simulink model "MeUn_VD"  (R2016b)
settings: configuration reference "CodeGenConfigSet" (kept outside this file)
values from neighbouring files (symbols this model uses):
  MeUn_bCrntClsdCtl_C = Calibration.Parameter    [init_MeUn_VD.m]
  MeUn_bFiterAct_C = Calibration.Parameter    [init_MeUn_VD.m]
  MeUn_bFuelTFit_C = Calibration.Parameter    [init_MeUn_VD.m]
  MeUn_CrntCtlIKi_C = Calibration.Parameter    [init_MeUn_VD.m]
  MeUn_CrntCtlIKiNeg_C = Calibration.Parameter    [init_MeUn_VD.m]
  MeUn_CrntCtlIKiPos_C = Calibration.Parameter    [init_MeUn_VD.m]
  MeUn_CrntCtlIWinNeg_C = Calibration.Parameter    [init_MeUn_VD.m]
  MeUn_CrntCtlIWinPos_C = Calibration.Parameter    [init_MeUn_VD.m]
  MeUn_facCrntCtlInit_CUR = Calibration.Parameter    [init_MeUn_VD.m]
  MeUn_facCrntCtlInit_CURX = Calibration.Parameter    [init_MeUn_VD.m]
  MeUn_facCrntCtlMax_C = Calibration.Parameter    [init_MeUn_VD.m]
  MeUn_facCrntCtlMin_C = Calibration.Parameter    [init_MeUn_VD.m]
  MeUn_facCrntOpenCtl_CUR = Calibration.Parameter    [init_MeUn_VD.m]
  MeUn_facCrntOpenCtl_CURX = Calibration.Parameter    [init_MeUn_VD.m]
  MeUn_facFlt1PT1_C = Calibration.Parameter    [init_MeUn_VD.m]
  MeUn_facFlt2PT1_C = Calibration.Parameter    [init_MeUn_VD.m]
  MeUn_iCnvFlowRate_CUR = Calibration.Parameter    [init_MeUn_VD.m]
  MeUn_iCnvFlowRate_CURX = Calibration.Parameter    [init_MeUn_VD.m]
  MeUn_iLin_CUR = Calibration.Parameter    [init_MeUn_VD.m]
  MeUn_iLin_CURX = Calibration.Parameter    [init_MeUn_VD.m]
  MeUn_iSetMin_C = Calibration.Parameter    [init_MeUn_VD.m]
  MeUn_stActrCtl_C = Calibration.Parameter    [init_MeUn_VD.m]
  MeUn_swtFrzICtl_C = Calibration.Parameter    [init_MeUn_VD.m]
  MeUn_swtVolt_C = Calibration.Parameter    [init_MeUn_VD.m]
  MeUn_tDefltTemp_C = Calibration.Parameter    [init_MeUn_VD.m]
  MeUn_tiCrntCtlInit_C = Calibration.Parameter    [init_MeUn_VD.m]
  MeUn_tiSRCMaxDefDeb_C = Calibration.Parameter    [init_MeUn_VD.m]
  MeUn_tiSRCMaxOKDeb_C = Calibration.Parameter    [init_MeUn_VD.m]
  MeUn_tiSRCMinDefDeb_C = Calibration.Parameter    [init_MeUn_VD.m]
  MeUn_tiSRCMinOKDeb_C = Calibration.Parameter    [init_MeUn_VD.m]
  MeUn_tTempInitThrsd_C = Calibration.Parameter    [init_MeUn_VD.m]
  MeUn_uSRCMax_C = Calibration.Parameter    [init_MeUn_VD.m]
  MeUn_uSRCMin_C = Calibration.Parameter    [init_MeUn_VD.m]
  MeUn_VoltLin_CUR = Calibration.Parameter    [init_MeUn_VD.m]
  MeUn_VoltLin_CURX = Calibration.Parameter    [init_MeUn_VD.m]
  SigTst_iMeUnCurrent_C = Calibration.Parameter    [init_MeUn_VD.m]
  SigTst_swtMeUnCurrent_C = Calibration.Parameter    [init_MeUn_VD.m]
undefined symbols (not defined in the file or in its folder): MeUn_VD_DT
libraries: CXLib x11, simulink x1
settings Model: Creator=Wollf  LastModifiedBy=liutao
settings ConfigSetRef: SourceLocation=Base Workspace

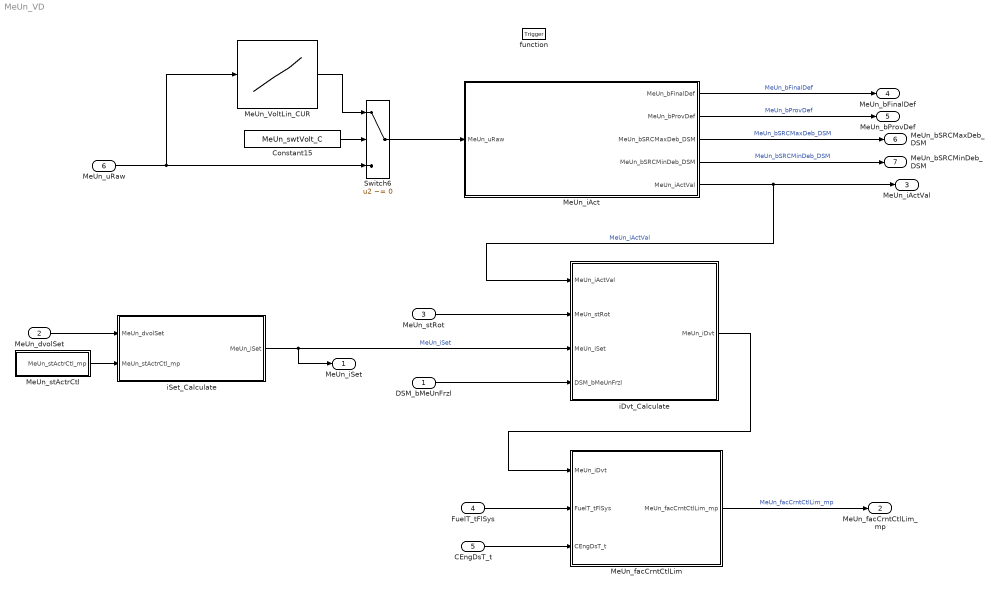
== system MeUn_VD ==
  DSM_bMeUnFrzl : Inport  Description=state of FId_MeUnFrzl  OutMin=0  OutMax=1  OutDataTypeStr=boolean
  MeUn_dvolSet : Inport  Tag=mm^3/s  Description=Setpoint value (volume flow) of rail pressure governing  Port=2  OutMin=-327670  OutMax=327670  OutDataTypeStr=FuelVol_mm3_s
  MeUn_stRot : Inport  Description=State of anchor rotation function of metering unit  Port=3  OutMin=0  OutMax=1  OutDataTypeStr=boolean
  FuelT_tFlSys : Inport  Tag=deg  Description=Fuel system temperature  Port=4  OutMin=-50  OutMax=200  OutDataTypeStr=Temp_deg
  CEngDsT_t : Inport  Tag=deg  Description=engine coolant temperature after filter  Port=5  OutMin=-200  OutMax=200  OutDataTypeStr=Temp_deg
  MeUn_uRaw : Inport  Tag=mv  Description=Raw value of meun  Port=6  OutMin=0  OutMax=5000  OutDataTypeStr=Ad_mv
  function : TriggerPort  TriggerType=function-call  VariantControl=Variant
  Constant15 : Constant  Value=MeUn_swtVolt_C
  MeUn_VoltLin_CUR : Lookup_n-D  NumberOfTableDimensions=1  BreakpointsForDimension1=MeUn_VoltLin_CURX  IndexSearchMethod=Linear search  BeginIndexSearchUsingPreviousIndexResult=on  UseOneInputPortForAllInputData=on  Table=MeUn_VoltLin_CUR  ExtrapMethod=Clip  UseLastTableValue=on  InternalRulePriority=Speed  OutDataTypeStr=Inherit: Inherit via back propagation  SaturateOnIntegerOverflow=on
  MeUn_facCrntCtlLim : Subsystem
  MeUn_iAct : Subsystem
  MeUn_stActrCtl : Subsystem
  Switch6 : Switch  Criteria=u2 ~= 0  InputSameDT=on
  iDvt_Calculate : Subsystem
  iSet_Calculate : Subsystem
  MeUn_iSet : Outport  Tag=mA  Description=Setpoint current for the metering unit  OutMin=-12000  OutMax=12000  OutDataTypeStr=Current_mA
  MeUn_facCrntCtlLim_mp : Outport  Description=Metering unit current control, I component  Port=2  OutMin=0  OutMax=15  OutDataTypeStr=Pid_Kp_Kd
  MeUn_iActVal : Outport  Tag=mA  Description=Current actual value of the analog intput  Port=3  OutMin=-12000  OutMax=12000  OutDataTypeStr=Current_mA
  MeUn_bFinalDef : Outport  Description=the final fault flag  Port=4  OutMin=0  OutMax=1  OutDataTypeStr=boolean
  MeUn_bProvDef : Outport  Description=the fault flag for the moment  Port=5  OutMin=0  OutMax=1  OutDataTypeStr=boolean
  MeUn_bSRCMaxDeb_DSM : Outport  Description=SRC High for metering unit voltage  Port=6  OutMin=0  OutMax=1  OutDataTypeStr=boolean
  MeUn_bSRCMinDeb_DSM : Outport  Description=SRC Low for metering unit voltage  Port=7  OutMin=0  OutMax=1  OutDataTypeStr=boolean
  wires:
  MeUn_stRot/1 -> iDvt_Calculate/2(MeUn_stRot)
  iDvt_Calculate/1(MeUn_iDvt) -> MeUn_facCrntCtlLim/1(MeUn_iDvt)
  MeUn_facCrntCtlLim/1(MeUn_facCrntCtlLim_mp) -> MeUn_facCrntCtlLim_mp/1  "MeUn_facCrntCtlLim_mp"
  DSM_bMeUnFrzl/1 -> iDvt_Calculate/4(DSM_bMeUnFrzl)
  FuelT_tFlSys/1 -> MeUn_facCrntCtlLim/2(FuelT_tFlSys)
  CEngDsT_t/1 -> MeUn_facCrntCtlLim/3(CEngDsT_t)
  Switch6/1 -> MeUn_iAct/1(MeUn_uRaw)
  MeUn_iAct/5(MeUn_iActVal) -> iDvt_Calculate/1(MeUn_iActVal), MeUn_iActVal/1  "MeUn_iActVal"
  MeUn_iAct/1(MeUn_bFinalDef) -> MeUn_bFinalDef/1  "MeUn_bFinalDef"
  MeUn_iAct/2(MeUn_bProvDef) -> MeUn_bProvDef/1  "MeUn_bProvDef"
  MeUn_iAct/3(MeUn_bSRCMaxDeb_DSM) -> MeUn_bSRCMaxDeb_DSM/1  "MeUn_bSRCMaxDeb_DSM"
  MeUn_iAct/4(MeUn_bSRCMinDeb_DSM) -> MeUn_bSRCMinDeb_DSM/1  "MeUn_bSRCMinDeb_DSM"
  iSet_Calculate/1(MeUn_iSet) -> iDvt_Calculate/3(MeUn_iSet), MeUn_iSet/1  "MeUn_iSet"
  MeUn_dvolSet/1 -> iSet_Calculate/1(MeUn_dvolSet)
  MeUn_stActrCtl/1(MeUn_stActrCtl_mp) -> iSet_Calculate/2(MeUn_stActrCtl_mp)
  Constant15/1 -> Switch6/2
  MeUn_uRaw/1 -> MeUn_VoltLin_CUR/1, Switch6/3
  MeUn_VoltLin_CUR/1 -> Switch6/1

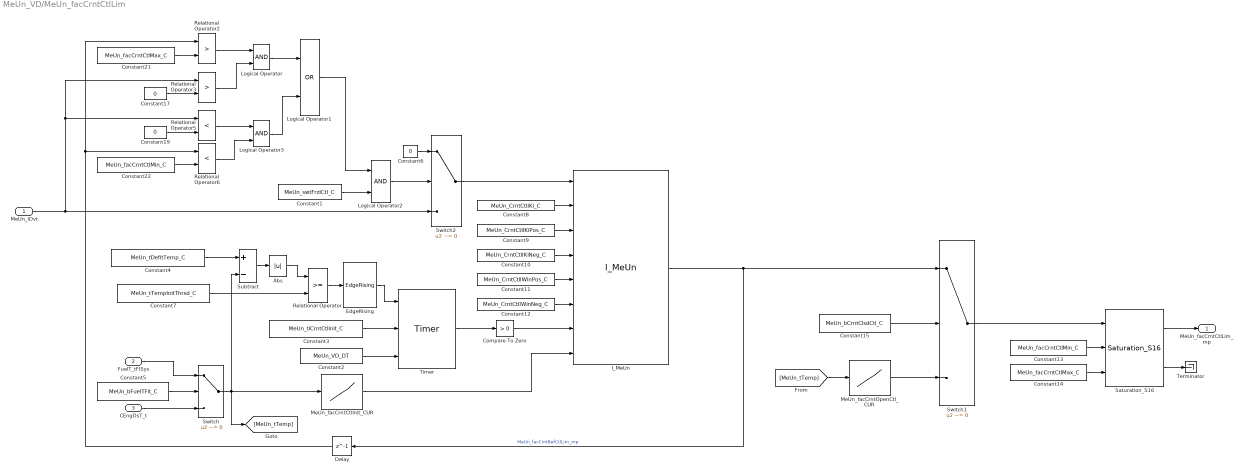
== system MeUn_VD/MeUn_facCrntCtlLim ==
  MeUn_iDvt : Inport
  FuelT_tFlSys : Inport  Port=2
  CEngDsT_t : Inport  Port=3
  Abs : Abs
  Compare To Zero : simulink/Logic and Bit Operations/Compare To Zero  relop=>  OutDataTypeStr=boolean
  Constant1 : Constant  Value=MeUn_swtFrzICtl_C
  Constant10 : Constant  Value=MeUn_CrntCtlIKiNeg_C
  Constant11 : Constant  Value=MeUn_CrntCtlIWinPos_C
  Constant12 : Constant  Value=MeUn_CrntCtlIWinNeg_C
  Constant13 : Constant  Value=MeUn_facCrntCtlMin_C
  Constant14 : Constant  Value=MeUn_facCrntCtlMax_C
  Constant15 : Constant  Value=MeUn_bCrntClsdCtl_C
  Constant17 : Constant  Value=0  OutDataTypeStr=Inherit: Inherit via back propagation  SampleTime=-1
  Constant19 : Constant  Value=0  OutDataTypeStr=Inherit: Inherit via back propagation  SampleTime=-1
  Constant2 : Constant  Value=MeUn_VD_DT
  Constant21 : Constant  Value=MeUn_facCrntCtlMax_C
  Constant22 : Constant  Value=MeUn_facCrntCtlMin_C
  Constant3 : Constant  Value=MeUn_tiCrntCtlInit_C
  Constant4 : Constant  Value=MeUn_tDefltTemp_C
  Constant5 : Constant  Value=MeUn_bFuelTFit_C
  Constant6 : Constant  Value=0  OutDataTypeStr=Inherit: Inherit via back propagation
  Constant7 : Constant  Value=MeUn_tTempInitThrsd_C
  Constant8 : Constant  Value=MeUn_CrntCtlIKi_C
  Constant9 : Constant  Value=MeUn_CrntCtlIKiPos_C
  Delay : Delay  DelayLength=1  InitialCondition=0
  EdgeRising : CXLib/EdgeRising
  I_MeUn : CXLib/I_MeUn
  Logical Operator : Logic  AllPortsSameDT=off  OutDataTypeStr=boolean
  Logical Operator1 : Logic  Operator=OR  OutDataTypeStr=boolean
  Logical Operator2 : Logic  AllPortsSameDT=off  OutDataTypeStr=boolean
  Logical Operator3 : Logic  AllPortsSameDT=off  OutDataTypeStr=boolean
  MeUn_facCrntCtlInit_CUR : Lookup_n-D  NumberOfTableDimensions=1  BreakpointsForDimension1=MeUn_facCrntCtlInit_CURX  Table=MeUn_facCrntCtlInit_CUR  TableDataTypeStr=Inherit: Inherit from 'Table data'  ExtrapMethod=Clip  InternalRulePriority=Speed  OutDataTypeStr=Inherit: Inherit from 'Table data'  RndMeth=Simplest
  MeUn_facCrntOpenCtl_CUR : Lookup_n-D  NumberOfTableDimensions=1  BreakpointsForDimension1=MeUn_facCrntOpenCtl_CURX  Table=MeUn_facCrntOpenCtl_CUR  TableDataTypeStr=Inherit: Inherit from 'Table data'  ExtrapMethod=Clip  InternalRulePriority=Speed  OutDataTypeStr=Inherit: Inherit from 'Table data'  RndMeth=Simplest
  Relational Operator : RelationalOperator  OutDataTypeStr=boolean  RndMeth=Simplest
  Relational Operator2 : RelationalOperator  Operator=>  OutDataTypeStr=boolean  RndMeth=Nearest  InputSameDT=on
  Relational Operator3 : RelationalOperator  Operator=>  OutDataTypeStr=boolean  RndMeth=Nearest  InputSameDT=on
  Relational Operator5 : RelationalOperator  Operator=<  OutDataTypeStr=boolean  RndMeth=Nearest  InputSameDT=on
  Relational Operator6 : RelationalOperator  Operator=<  OutDataTypeStr=boolean  RndMeth=Nearest  InputSameDT=on
  Saturation_S16 : CXLib/Saturation_S16
  Subtract : Sum  Inputs=+-
  Switch : Switch  Criteria=u2 ~= 0
  Switch1 : Switch  Criteria=u2 ~= 0
  Switch2 : Switch  Criteria=u2 ~= 0  InputSameDT=on
  Terminator : Terminator
  Timer : CXLib/Timer
  MeUn_facCrntCtlLim_mp : Outport
  wires:
  I_MeUn/1 -> Delay/1, Switch1/1  "MeUn_facCrntBefCtlLim_mp"
  Constant13/1 -> Saturation_S16/2
  Constant14/1 -> Saturation_S16/3
  Saturation_S16/1 -> MeUn_facCrntCtlLim_mp/1
  Saturation_S16/2 -> Terminator/1
  Constant9/1 -> I_MeUn/3
  Constant10/1 -> I_MeUn/4
  Constant11/1 -> I_MeUn/5
  Constant12/1 -> I_MeUn/6
  Constant8/1 -> I_MeUn/2
  Logical Operator3/1 -> Logical Operator1/2
  Logical Operator/1 -> Logical Operator1/1
  Constant21/1 -> Relational Operator2/2
  Constant17/1 -> Relational Operator3/2
  MeUn_iDvt/1 -> Switch2/3, Relational Operator3/1, Relational Operator5/1
  Relational Operator2/1 -> Logical Operator/1
  Relational Operator3/1 -> Logical Operator/2
  Constant19/1 -> Relational Operator5/2
  Relational Operator5/1 -> Logical Operator3/1
  Relational Operator6/1 -> Logical Operator3/2
  Constant22/1 -> Relational Operator6/2
  Switch2/1 -> I_MeUn/1
  Constant6/1 -> Switch2/1
  Constant1/1 -> Logical Operator2/2
  Logical Operator2/1 -> Switch2/2
  Logical Operator1/1 -> Logical Operator2/1
  Delay/1 -> Relational Operator6/1, Relational Operator2/1
  Constant2/1 -> Timer/3
  Constant3/1 -> Timer/2
  EdgeRising/1 -> Timer/1
  FuelT_tFlSys/1 -> Switch/1
  CEngDsT_t/1 -> Switch/3
  Constant5/1 -> Switch/2
  Switch/1 -> [MeUn_tTemp], Subtract/2, MeUn_facCrntCtlInit_CUR/1
  MeUn_facCrntCtlInit_CUR/1 -> I_MeUn/8
  Timer/1 -> Compare To Zero/1
  Constant4/1 -> Subtract/1
  Subtract/1 -> Abs/1
  Relational Operator/1 -> EdgeRising/1
  Abs/1 -> Relational Operator/1
  Constant7/1 -> Relational Operator/2
  Compare To Zero/1 -> I_MeUn/7
  Switch1/1 -> Saturation_S16/1
  MeUn_facCrntOpenCtl_CUR/1 -> Switch1/3
  Constant15/1 -> Switch1/2
  [MeUn_tTemp] -> MeUn_facCrntOpenCtl_CUR/1

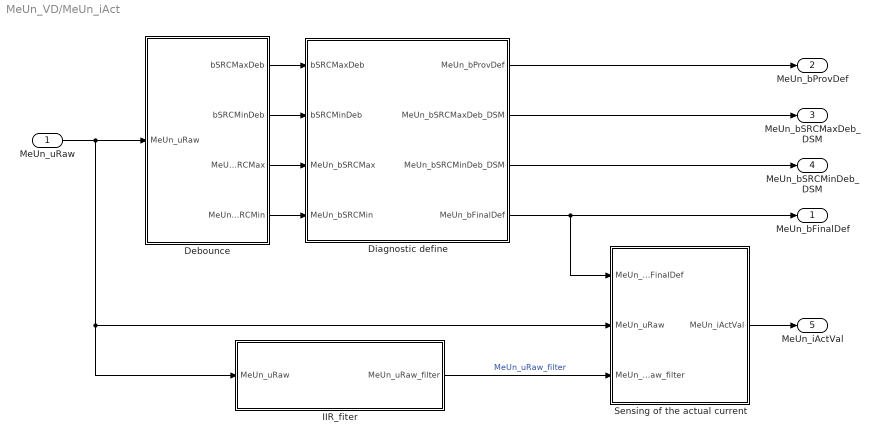
== system MeUn_VD/MeUn_iAct ==
  MeUn_uRaw : Inport
  Debounce : Subsystem
  Diagnostic define : Subsystem
  IIR_fiter : Subsystem  Tag=FilterWizardSubSystem
      settings: ErrorFcn=dspFilterRealizedInBasicElemsAlgLoopErrFcnCallback
  Sensing of the actual current : Subsystem
  MeUn_bFinalDef : Outport
  MeUn_bProvDef : Outport  Port=2
  MeUn_bSRCMaxDeb_DSM : Outport  Port=3
  MeUn_bSRCMinDeb_DSM : Outport  Port=4
  MeUn_iActVal : Outport  Port=5
  wires:
  Sensing of the actual current/1(MeUn_iActVal) -> MeUn_iActVal/1
  MeUn_uRaw/1 -> IIR_fiter/1(MeUn_uRaw), Sensing of the actual current/2(MeUn_uRaw), Debounce/1(MeUn_uRaw)
  Debounce/1(bSRCMaxDeb) -> Diagnostic define/1(bSRCMaxDeb)
  Debounce/2(bSRCMinDeb) -> Diagnostic define/2(bSRCMinDeb)
  Diagnostic define/1(MeUn_bProvDef) -> MeUn_bProvDef/1
  Debounce/3(MeUn_bSRCMax) -> Diagnostic define/3(MeUn_bSRCMax)
  Debounce/4(MeUn_bSRCMin) -> Diagnostic define/4(MeUn_bSRCMin)
  Diagnostic define/4(MeUn_bFinalDef) -> MeUn_bFinalDef/1, Sensing of the actual current/1(MeUn_bFinalDef)
  Diagnostic define/2(MeUn_bSRCMaxDeb_DSM) -> MeUn_bSRCMaxDeb_DSM/1
  Diagnostic define/3(MeUn_bSRCMinDeb_DSM) -> MeUn_bSRCMinDeb_DSM/1
  IIR_fiter/1(MeUn_uRaw_filter) -> Sensing of the actual current/3(MeUn_uRaw_filter)  "MeUn_uRaw_filter"

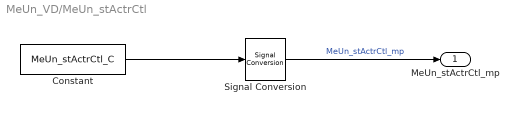
== system MeUn_VD/MeUn_stActrCtl ==
  Constant : Constant  Value=MeUn_stActrCtl_C
  Signal Conversion : SignalConversion  OverrideOpt=off
  MeUn_stActrCtl_mp : Outport
  wires:
  Constant/1 -> Signal Conversion/1
  Signal Conversion/1 -> MeUn_stActrCtl_mp/1  "MeUn_stActrCtl_mp"

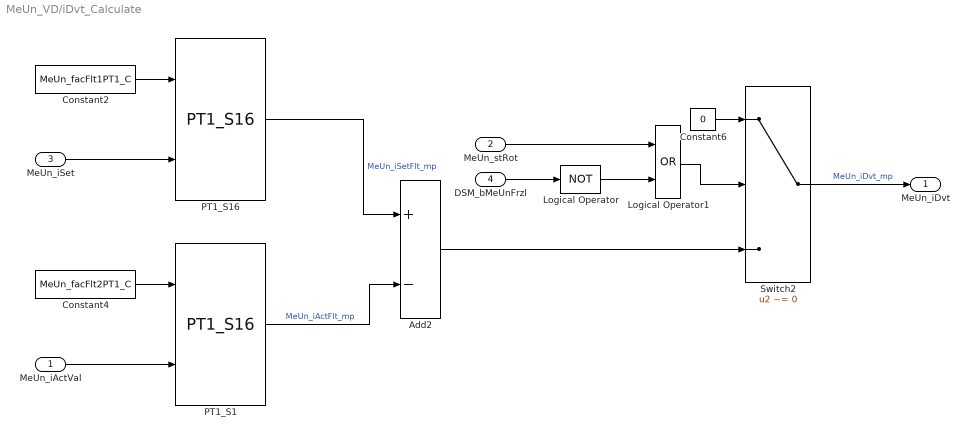
== system MeUn_VD/iDvt_Calculate ==
  MeUn_iActVal : Inport
  MeUn_stRot : Inport  Port=2
  MeUn_iSet : Inport  Port=3
  DSM_bMeUnFrzl : Inport  Port=4
  Add2 : Sum  Inputs=+-  OutDataTypeStr=Inherit: Inherit via back propagation  InputSameDT=on
  Constant2 : Constant  Value=MeUn_facFlt1PT1_C
  Constant4 : Constant  Value=MeUn_facFlt2PT1_C
  Constant6 : Constant  Value=0  OutDataTypeStr=Inherit: Inherit via back propagation
  Logical Operator : Logic  Operator=NOT  AllPortsSameDT=off  OutDataTypeStr=boolean
  Logical Operator1 : Logic  Operator=OR  OutDataTypeStr=boolean
  PT1_S1 : CXLib/PT1_S16
  PT1_S16 : CXLib/PT1_S16
  Switch2 : Switch  Criteria=u2 ~= 0  InputSameDT=on
  MeUn_iDvt : Outport
  wires:
  Add2/1 -> Switch2/3
  Logical Operator1/1 -> Switch2/2
  Constant6/1 -> Switch2/1
  Switch2/1 -> MeUn_iDvt/1  "MeUn_iDvt_mp"
  Logical Operator/1 -> Logical Operator1/2
  DSM_bMeUnFrzl/1 -> Logical Operator/1
  PT1_S16/1 -> Add2/1  "MeUn_iSetFlt_mp"
  PT1_S1/1 -> Add2/2  "MeUn_iActFlt_mp"
  MeUn_iActVal/1 -> PT1_S1/2
  Constant2/1 -> PT1_S16/1
  Constant4/1 -> PT1_S1/1
  MeUn_stRot/1 -> Logical Operator1/1
  MeUn_iSet/1 -> PT1_S16/2

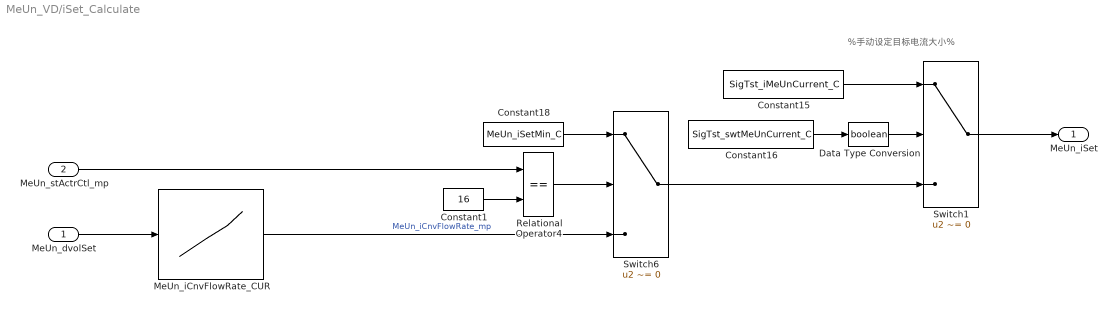
== system MeUn_VD/iSet_Calculate ==
  note: %手动设定目标电流大小%
  MeUn_dvolSet : Inport
  MeUn_stActrCtl_mp : Inport  Port=2
  Constant1 : Constant  Value=16  OutDataTypeStr=Inherit: Inherit via back propagation
  Constant15 : Constant  Value=SigTst_iMeUnCurrent_C
  Constant16 : Constant  Value=SigTst_swtMeUnCurrent_C
  Constant18 : Constant  Value=MeUn_iSetMin_C
  Data Type Conversion : DataTypeConversion  OutDataTypeStr=boolean
  MeUn_iCnvFlowRate_CUR : Lookup_n-D  NumberOfTableDimensions=1  BreakpointsForDimension1=MeUn_iCnvFlowRate_CURX  IndexSearchMethod=Linear search  BeginIndexSearchUsingPreviousIndexResult=on  UseOneInputPortForAllInputData=on  Table=MeUn_iCnvFlowRate_CUR  ExtrapMethod=Clip  UseLastTableValue=on  InternalRulePriority=Speed  OutDataTypeStr=Inherit: Inherit via back propagation  SaturateOnIntegerOverflow=on
  Relational Operator4 : RelationalOperator  Operator===  OutDataTypeStr=boolean  RndMeth=Nearest  InputSameDT=on
  Switch1 : Switch  Criteria=u2 ~= 0  InputSameDT=on
  Switch6 : Switch  Criteria=u2 ~= 0  InputSameDT=on
  MeUn_iSet : Outport
  wires:
  MeUn_dvolSet/1 -> MeUn_iCnvFlowRate_CUR/1
  MeUn_iCnvFlowRate_CUR/1 -> Switch6/3  "MeUn_iCnvFlowRate_mp"
  MeUn_stActrCtl_mp/1 -> Relational Operator4/1
  Constant1/1 -> Relational Operator4/2
  Relational Operator4/1 -> Switch6/2
  Constant18/1 -> Switch6/1
  Switch6/1 -> Switch1/3
  Constant16/1 -> Data Type Conversion/1
  Constant15/1 -> Switch1/1
  Data Type Conversion/1 -> Switch1/2
  Switch1/1 -> MeUn_iSet/1

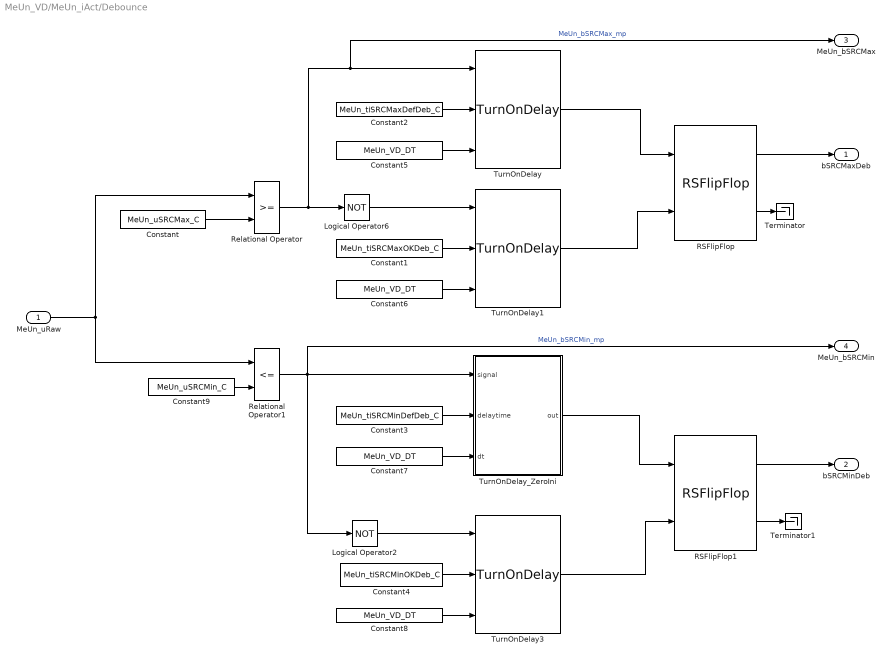
== system MeUn_VD/MeUn_iAct/Debounce ==
  MeUn_uRaw : Inport
  Constant : Constant  Value=MeUn_uSRCMax_C
  Constant1 : Constant  Value=MeUn_tiSRCMaxOKDeb_C
  Constant2 : Constant  Value=MeUn_tiSRCMaxDefDeb_C
  Constant3 : Constant  Value=MeUn_tiSRCMinDefDeb_C
  Constant4 : Constant  Value=MeUn_tiSRCMinOKDeb_C
  Constant{5..8} (4 alike) : Constant  Value=MeUn_VD_DT  OutDataTypeStr=Debounce_ms
  Constant9 : Constant  Value=MeUn_uSRCMin_C
  Logical Operator2 : Logic  Operator=NOT  AllPortsSameDT=off  OutDataTypeStr=boolean
  Logical Operator6 : Logic  Operator=NOT  AllPortsSameDT=off  OutDataTypeStr=boolean
  RSFlipFlop : CXLib/RSFlipFlop
  RSFlipFlop1 : CXLib/RSFlipFlop
  Relational Operator : RelationalOperator  OutDataTypeStr=boolean  RndMeth=Nearest  InputSameDT=on
  Relational Operator1 : RelationalOperator  Operator=<=  OutDataTypeStr=boolean  RndMeth=Nearest  InputSameDT=on
  Terminator : Terminator
  Terminator1 : Terminator
  TurnOnDelay : CXLib/TurnOnDelay
  TurnOnDelay1 : CXLib/TurnOnDelay
  TurnOnDelay3 : CXLib/TurnOnDelay
  TurnOnDelay_ZeroIni : Subsystem  RTWFcnName=lib_turn_on_delay  RTWFileName=service_library  mask(TurnOnDelay){}
      mask help:
      | 开启延迟：输入信号从0-->1时延时一定时间，保证信号确认。
      |
      | In1（boolean）: signal;
      | In2（Debounce_ms）: delaytime,延时时间（0~4294967295ms）;
      | In3（Debounce_ms）: dt，采样时间；
      |
      | Out1（boolean）: out
      mask Display:
      | %disp('TurnOn\nDelay')
      | image('TurnOnDelay.jpg')
  bSRCMaxDeb : Outport
  bSRCMinDeb : Outport  Port=2
  MeUn_bSRCMax : Outport  Port=3
  MeUn_bSRCMin : Outport  Port=4
  wires:
  RSFlipFlop1/1 -> bSRCMinDeb/1
  RSFlipFlop/1 -> bSRCMaxDeb/1
  TurnOnDelay1/1 -> RSFlipFlop/2
  Constant3/1 -> TurnOnDelay_ZeroIni/2(delaytime)
  Constant1/1 -> TurnOnDelay1/2
  Constant2/1 -> TurnOnDelay/2
  TurnOnDelay/1 -> RSFlipFlop/1
  Logical Operator6/1 -> TurnOnDelay1/1
  TurnOnDelay_ZeroIni/1(out) -> RSFlipFlop1/1
  TurnOnDelay3/1 -> RSFlipFlop1/2
  Constant4/1 -> TurnOnDelay3/2
  RSFlipFlop/2 -> Terminator/1
  RSFlipFlop1/2 -> Terminator1/1
  Constant5/1 -> TurnOnDelay/3
  Constant6/1 -> TurnOnDelay1/3
  Constant7/1 -> TurnOnDelay_ZeroIni/3(dt)
  Constant8/1 -> TurnOnDelay3/3
  Constant/1 -> Relational Operator/2
  Relational Operator/1 -> MeUn_bSRCMax/1, TurnOnDelay/1, Logical Operator6/1  "MeUn_bSRCMax_mp"
  Constant9/1 -> Relational Operator1/2
  Relational Operator1/1 -> MeUn_bSRCMin/1, Logical Operator2/1, TurnOnDelay_ZeroIni/1(signal)  "MeUn_bSRCMin_mp"
  Logical Operator2/1 -> TurnOnDelay3/1
  MeUn_uRaw/1 -> Relational Operator/1, Relational Operator1/1

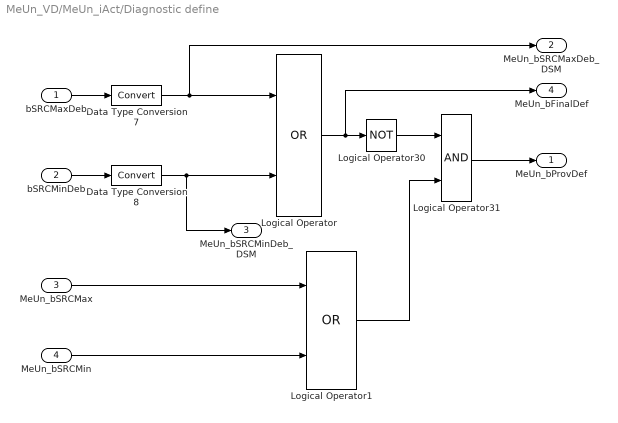
== system MeUn_VD/MeUn_iAct/Diagnostic define ==
  bSRCMaxDeb : Inport
  bSRCMinDeb : Inport  Port=2
  MeUn_bSRCMax : Inport  Port=3
  MeUn_bSRCMin : Inport  Port=4
  Data Type Conversion7 : DataTypeConversion
  Data Type Conversion8 : DataTypeConversion
  Logical Operator : Logic  Operator=OR  AllPortsSameDT=off  OutDataTypeStr=boolean
  Logical Operator1 : Logic  Operator=OR  AllPortsSameDT=off  OutDataTypeStr=boolean
  Logical Operator30 : Logic  Operator=NOT  AllPortsSameDT=off  OutDataTypeStr=boolean
  Logical Operator31 : Logic  AllPortsSameDT=off  OutDataTypeStr=boolean
  MeUn_bProvDef : Outport
  MeUn_bSRCMaxDeb_DSM : Outport  Port=2
  MeUn_bSRCMinDeb_DSM : Outport  Port=3
  MeUn_bFinalDef : Outport  Port=4
  wires:
  bSRCMaxDeb/1 -> Data Type Conversion7/1
  bSRCMinDeb/1 -> Data Type Conversion8/1
  Logical Operator/1 -> Logical Operator30/1, MeUn_bFinalDef/1
  Data Type Conversion7/1 -> Logical Operator/1, MeUn_bSRCMaxDeb_DSM/1
  Data Type Conversion8/1 -> Logical Operator/2, MeUn_bSRCMinDeb_DSM/1
  Logical Operator31/1 -> MeUn_bProvDef/1
  Logical Operator30/1 -> Logical Operator31/1
  Logical Operator1/1 -> Logical Operator31/2
  MeUn_bSRCMax/1 -> Logical Operator1/1
  MeUn_bSRCMin/1 -> Logical Operator1/2

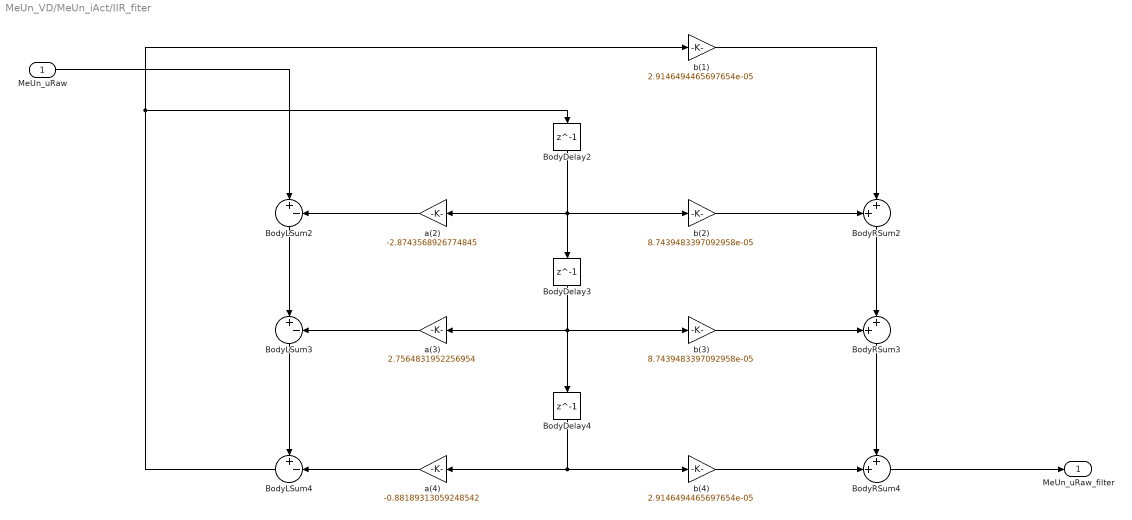
== system MeUn_VD/MeUn_iAct/IIR_fiter ==
  MeUn_uRaw : Inport
  BodyDelay2 : Delay  DelayLength=1  InitialCondition=0
  BodyDelay3 : Delay  DelayLength=1  InitialCondition=0
  BodyDelay4 : Delay  DelayLength=1  InitialCondition=0
  BodyLSum2 : Sum  Inputs=|+-  OutDataTypeStr=fixdt(1,32,5)  RndMeth=Nearest  SaturateOnIntegerOverflow=on
  BodyLSum3 : Sum  Inputs=|+-  OutDataTypeStr=fixdt(1,32,10)  RndMeth=Nearest  SaturateOnIntegerOverflow=on
  BodyLSum4 : Sum  Inputs=+-|  OutDataTypeStr=fixdt(1,32,7)  RndMeth=Nearest  SaturateOnIntegerOverflow=on
  BodyRSum2 : Sum  Inputs=++|  OutDataTypeStr=fixdt(1,32,20)  RndMeth=Nearest  SaturateOnIntegerOverflow=on
  BodyRSum3 : Sum  Inputs=++|  OutDataTypeStr=fixdt(1,32,19)  RndMeth=Nearest  SaturateOnIntegerOverflow=on
  BodyRSum4 : Sum  Inputs=++|  OutDataTypeStr=Inherit: Inherit via back propagation  RndMeth=Nearest  SaturateOnIntegerOverflow=on
  a(2) : Gain  Gain=-2.8743568926774845  ParamDataTypeStr=fixdt(1,32,29)  OutDataTypeStr=fixdt(1,32,5)  RndMeth=Nearest  SaturateOnIntegerOverflow=on
  a(3) : Gain  Gain=2.7564831952256954  ParamDataTypeStr=fixdt(1,32,29)  OutDataTypeStr=fixdt(1,32,5)  RndMeth=Nearest  SaturateOnIntegerOverflow=on
  a(4) : Gain  Gain=-0.88189313059248542  ParamDataTypeStr=fixdt(1,32,31)  OutDataTypeStr=fixdt(1,32,7)  RndMeth=Nearest  SaturateOnIntegerOverflow=on
  b(1) : Gain  Gain=2.9146494465697654e-05  ParamDataTypeStr=fixdt(1,32,46)  OutDataTypeStr=fixdt(1,32,22)  RndMeth=Nearest  SaturateOnIntegerOverflow=on
  b(2) : Gain  Gain=8.7439483397092958e-05  ParamDataTypeStr=fixdt(1,32,44)  OutDataTypeStr=fixdt(1,32,20)  RndMeth=Nearest  SaturateOnIntegerOverflow=on
  b(3) : Gain  Gain=8.7439483397092958e-05  ParamDataTypeStr=fixdt(1,32,44)  OutDataTypeStr=fixdt(1,32,20)  RndMeth=Nearest  SaturateOnIntegerOverflow=on
  b(4) : Gain  Gain=2.9146494465697654e-05  ParamDataTypeStr=fixdt(1,32,46)  OutDataTypeStr=fixdt(1,32,22)  RndMeth=Nearest  SaturateOnIntegerOverflow=on
  MeUn_uRaw_filter : Outport
  wires:
  b(1)/1 -> BodyRSum2/2
  MeUn_uRaw/1 -> BodyLSum2/1
  BodyLSum2/1 -> BodyLSum3/1
  a(2)/1 -> BodyLSum2/2
  BodyDelay2/1 -> a(2)/1, b(2)/1, BodyDelay3/1
  b(2)/1 -> BodyRSum2/1
  BodyRSum2/1 -> BodyRSum3/2
  BodyLSum3/1 -> BodyLSum4/1
  a(3)/1 -> BodyLSum3/2
  BodyDelay3/1 -> a(3)/1, b(3)/1, BodyDelay4/1
  b(3)/1 -> BodyRSum3/1
  BodyRSum3/1 -> BodyRSum4/1
  BodyLSum4/1 -> b(1)/1, BodyDelay2/1
  a(4)/1 -> BodyLSum4/2
  BodyDelay4/1 -> a(4)/1, b(4)/1
  b(4)/1 -> BodyRSum4/2
  BodyRSum4/1 -> MeUn_uRaw_filter/1

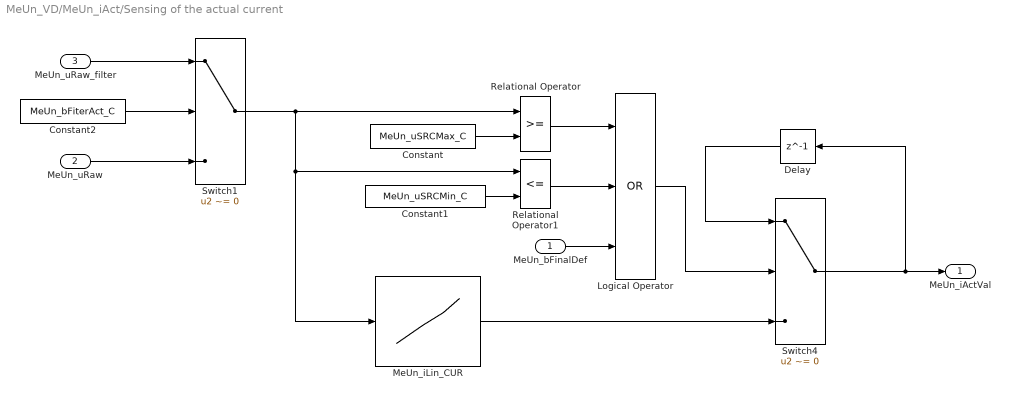
== system MeUn_VD/MeUn_iAct/Sensing of the actual current ==
  MeUn_bFinalDef : Inport
  MeUn_uRaw : Inport  Port=2
  MeUn_uRaw_filter : Inport  Port=3
  Constant : Constant  Value=MeUn_uSRCMax_C
  Constant1 : Constant  Value=MeUn_uSRCMin_C
  Constant2 : Constant  Value=MeUn_bFiterAct_C
  Delay : Delay  DelayLength=1  InitialCondition=0
  Logical Operator : Logic  Operator=OR  Inputs=3  OutDataTypeStr=boolean
  MeUn_iLin_CUR : Lookup_n-D  NumberOfTableDimensions=1  BreakpointsForDimension1=MeUn_iLin_CURX  IndexSearchMethod=Linear search  BeginIndexSearchUsingPreviousIndexResult=on  UseOneInputPortForAllInputData=on  Table=MeUn_iLin_CUR  ExtrapMethod=Clip  UseLastTableValue=on  InternalRulePriority=Speed  OutDataTypeStr=Inherit: Inherit via back propagation  SaturateOnIntegerOverflow=on
  Relational Operator : RelationalOperator  OutDataTypeStr=boolean  RndMeth=Nearest  InputSameDT=on
  Relational Operator1 : RelationalOperator  Operator=<=  OutDataTypeStr=boolean  RndMeth=Nearest  InputSameDT=on
  Switch1 : Switch  Criteria=u2 ~= 0  InputSameDT=on
  Switch4 : Switch  Criteria=u2 ~= 0  InputSameDT=on
  MeUn_iActVal : Outport
  wires:
  MeUn_bFinalDef/1 -> Logical Operator/3
  MeUn_iLin_CUR/1 -> Switch4/3
  Switch4/1 -> Delay/1, MeUn_iActVal/1
  Delay/1 -> Switch4/1
  Logical Operator/1 -> Switch4/2
  Relational Operator/1 -> Logical Operator/1
  Relational Operator1/1 -> Logical Operator/2
  Constant1/1 -> Relational Operator1/2
  Constant/1 -> Relational Operator/2
  Switch1/1 -> MeUn_iLin_CUR/1, Relational Operator1/1, Relational Operator/1
  MeUn_uRaw_filter/1 -> Switch1/1
  MeUn_uRaw/1 -> Switch1/3
  Constant2/1 -> Switch1/2

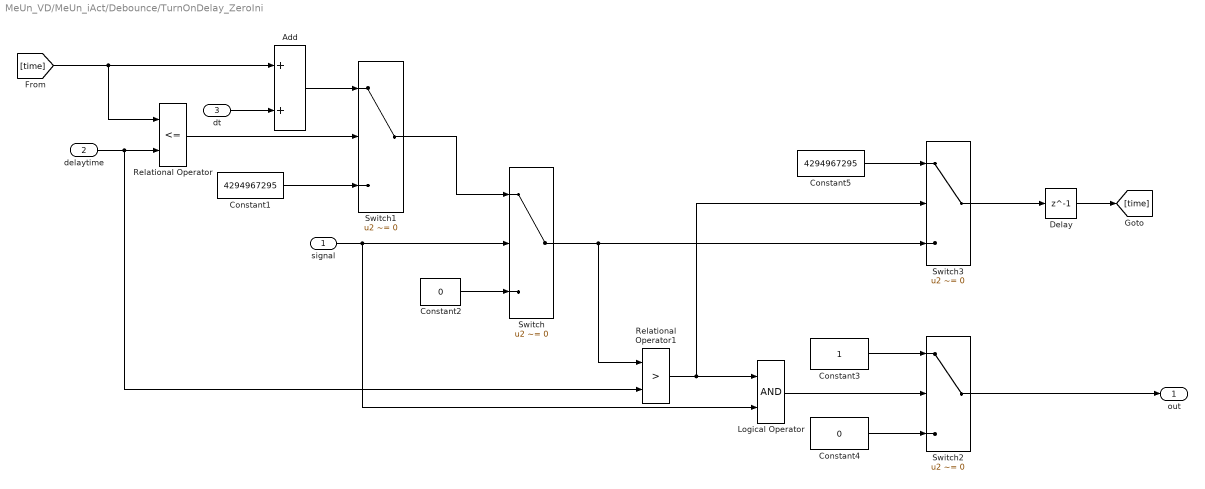
== system MeUn_VD/MeUn_iAct/Debounce/TurnOnDelay_ZeroIni ==
  signal : Inport  OutDataTypeStr=boolean
  delaytime : Inport  Port=2
  dt : Inport  Port=3
  Add : Sum  SaturateOnIntegerOverflow=on  InputSameDT=on
  Constant1 : Constant  Value=4294967295  OutDataTypeStr=Inherit: Inherit via back propagation
  Constant2 : Constant  Value=0  OutDataTypeStr=Inherit: Inherit via back propagation
  Constant3 : Constant  OutDataTypeStr=boolean
  Constant4 : Constant  Value=0  OutDataTypeStr=boolean
  Constant5 : Constant  Value=4294967295  OutDataTypeStr=Inherit: Inherit via back propagation
  Delay : Delay  DelayLength=1  InitialCondition=0  StateName=time
      settings: AttributesFormatString=InitialValue=%<InitialCondition>
  Logical Operator : Logic  OutDataTypeStr=boolean
  Relational Operator : RelationalOperator  Operator=<=  OutDataTypeStr=boolean  RndMeth=Nearest  InputSameDT=on
  Relational Operator1 : RelationalOperator  Operator=>  OutDataTypeStr=boolean  RndMeth=Nearest  InputSameDT=on
  Switch : Switch  Criteria=u2 ~= 0  SaturateOnIntegerOverflow=on  InputSameDT=on
  Switch1 : Switch  Criteria=u2 ~= 0  SaturateOnIntegerOverflow=on  InputSameDT=on
  Switch2 : Switch  Criteria=u2 ~= 0  RndMeth=Round  SaturateOnIntegerOverflow=on  InputSameDT=on
  Switch3 : Switch  Criteria=u2 ~= 0  RndMeth=Round  SaturateOnIntegerOverflow=on  InputSameDT=on
  out : Outport  OutDataTypeStr=boolean
  wires:
  Delay/1 -> [time]
  Switch3/1 -> Delay/1
  Constant5/1 -> Switch3/1
  Switch/1 -> Switch3/3, Relational Operator1/1
  Switch2/1 -> out/1
  Constant4/1 -> Switch2/3
  Constant3/1 -> Switch2/1
  Logical Operator/1 -> Switch2/2
  Relational Operator1/1 -> Logical Operator/1, Switch3/2
  Constant2/1 -> Switch/3
  Constant1/1 -> Switch1/3
  dt/1 -> Add/2
  [time] -> Add/1, Relational Operator/1
  Add/1 -> Switch1/1
  Relational Operator/1 -> Switch1/2
  delaytime/1 -> Relational Operator/2, Relational Operator1/2
  Switch1/1 -> Switch/1
  signal/1 -> Switch/2, Logical Operator/2
